simulink model "testForklift_hw"  (R2020b)
settings: Solver=FixedStepAuto  StartTime=0.0  StopTime=30  FixedStep=TS  RelTol=1e-3  EnableMultiTasking=on
model workspace (MAT data in the model file):
  TS = 0.01
libraries: arduinomotorcarrierlib x1
settings Model: SimulationMode=external  SILPILModeSetting=veronly  ExtModeTrigDuration=2  Creator=jmodiset  LastModifiedBy=arunkumar
settings DataIOCC: ReturnWorkspaceOutputs=off
settings OptimizationCC: PassReuseOutputArgsThreshold=0  MaxStackSize=64
settings DebuggingCC: UnderspecifiedInitializationDetection=Classic  MergeDetectMultiDrivingBlocksExec=none  ParameterTunabilityLossMsg=error  ArithmeticOperatorsInVariantConditions=warning
settings HardwareCC: ProdBitPerPointer=32  ProdBitPerSizeT=32  ProdBitPerPtrDiffT=32  ProdLargestAtomicInteger=Long  ProdLargestAtomicFloat=Double  ProdWordSize=32  ProdHWDeviceType=ARM Compatible->ARM Cortex  UseEmbeddedCoderFeatures=off  UseSimulinkCoderFeatures=off
settings SFSimCC: SimUseLocalCustomCode=off  MATLABDynamicMemAlloc=off  CustomCodeUndefinedFunction=UseInterfaceOnly
settings RTWCC: Description=Embedded Coder  SystemTargetFile=ert.tlc  HardwareBoard=Arduino Nano 33 IoT  TemplateMakefile=ert_default_tmf  RTWUseLocalCustomCode=off  Toolchain=Arduino ARM  BuildConfiguration=Faster Runs
settings CodeAppCC: ForceParamTrailComments=on  OperatorAnnotations=on
settings ERTTargetCC: ERTCustomFileBanners=off  SupportContinuousTime=on  SupportNonInlinedSFcns=on  RemoveResetFunc=off  SupportVariableSizeSignals=on  ModelStepFunctionPrototypeControlCompliant=off  ExtModeStaticAllocSize=8192

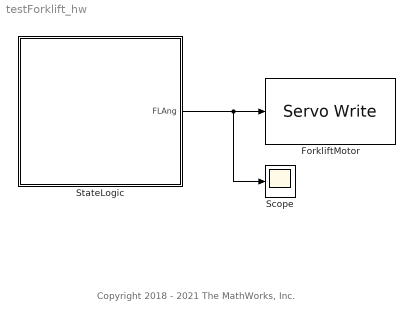
== system testForklift_hw ==
  note: Copyright 2018 - 2021 The MathWorks, Inc.
  ForkliftMotor : arduinomotorcarrierlib/Servo Write  SlaveAddress=uint8( hex2dec( '66' ) )  blockPlatform=ARDUINO  MotorNumber=3  MotorCarrierPWMFreq=100
      settings: SourceProductName=Simulink Support for Arduino MKR Motor Carrier
  Scope : Scope
  StateLogic : Stateflow chart  TreatAsAtomicUnit=on
  wires:
  StateLogic/1(FLAng) -> Scope/1, ForkliftMotor/1

== stateflow chart testForklift_hw/StateLogic ==
  state Start
    entry:
    FLAng = 125;
  state DropForklift
    entry, during, exit:
    FLAng = FLAng-0.5;
  state LiftForklift
    en, du, ex:
    FLAng = FLAng+0.5;
  state DoNothing1
    en, du, ex:
  (default) -> Start
  Start -> DropForklift : after(1,sec)
  DropForklift -> (junction 149) : [FLAng < 0.5]
  (junction 149) -> LiftForklift : after(1,sec)
  LiftForklift -> DoNothing1 : [FLAng > 124.5]
  data: FLAng output
